simulink model "TestMassAccelerometer_NonlinearModel_LQR_Simulink2017"  (R2018b)
settings: Solver=ode4  StartTime=0.0  StopTime=SIM_TIME  FixedStep=STEP_SIZE  RelTol=1e-3
undefined symbols (not defined in the file): A0, A1, c1, c2, f1, f2, f3, f4, f5, f6, g, Iss, K_lqr_fs, K_lqr_int, m, STEP_TIME, Ts, Vss, x0, x0_int, X_ref, Xss
settings Model: Creator=Roberto  LastModifiedBy=Roberto
settings SFSimCC: SimUseLocalCustomCode=off
settings RTWCC: RTWUseLocalCustomCode=off
settings CodeAppCC: StateflowObjectComments=on

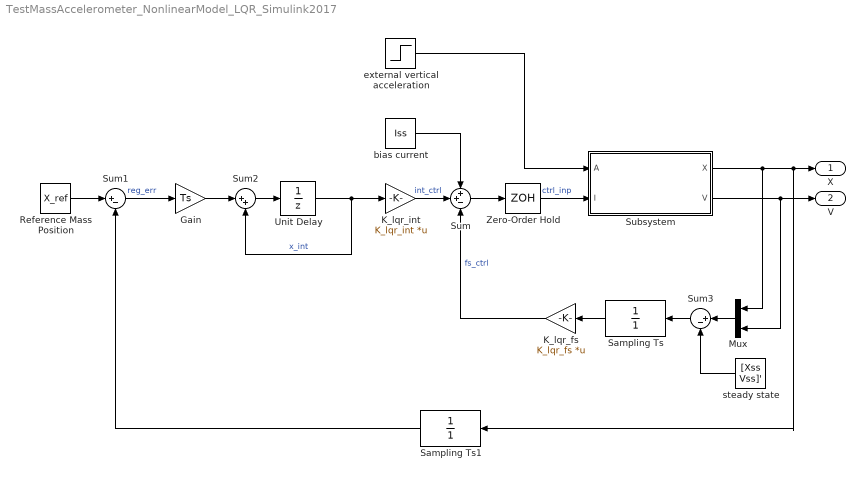
== system TestMassAccelerometer_NonlinearModel_LQR_Simulink2017 ==
  Gain : Gain  Gain=Ts
  K_lqr_fs : Gain  Gain=K_lqr_fs  Multiplication=Matrix(K*u) (u vector)
  K_lqr_int : Gain  Gain=K_lqr_int  Multiplication=Matrix(K*u) (u vector)
  Mux : Mux  Inputs=2
  Reference Mass Position : Constant  Value=X_ref
  Sampling Ts : DiscreteTransferFcn  Denominator=[1]  SampleTime=Ts
  Sampling Ts1 : DiscreteTransferFcn  Denominator=[1]  SampleTime=Ts
  Subsystem : Subsystem
  Sum : Sum  Inputs=++-
  Sum1 : Sum  Inputs=|+-
  Sum2 : Sum  Inputs=|++
  Sum3 : Sum  Inputs=|+-
  Unit Delay : UnitDelay  InitialCondition=x0_int  SampleTime=Ts
  Zero-Order Hold : ZeroOrderHold  SampleTime=Ts
  bias current : Constant  Value=Iss
  external vertical acceleration : Step  Time=STEP_TIME  Before=A0  After=A1  SampleTime=0
  steady state : Constant  Value=[Xss Vss]'
  X : Outport
  V : Outport  Port=2
  wires:
  Zero-Order Hold/1 -> Subsystem/2(I)  "ctrl_inp"
  Subsystem/2(V) -> Mux/2, V/1
  Sampling Ts/1 -> K_lqr_fs/1
  Sum/1 -> Zero-Order Hold/1
  K_lqr_fs/1 -> Sum/3  "fs_ctrl"
  Reference Mass Position/1 -> Sum1/1
  Subsystem/1(X) -> Mux/1, Sampling Ts1/1, X/1
  Sum2/1 -> Unit Delay/1
  Sum1/1 -> Gain/1  "reg_err"
  Unit Delay/1 -> Sum2/2, K_lqr_int/1  "x_int"
  K_lqr_int/1 -> Sum/2  "int_ctrl"
  bias current/1 -> Sum/1
  Sum3/1 -> Sampling Ts/1
  Mux/1 -> Sum3/1
  steady state/1 -> Sum3/2
  external vertical acceleration/1 -> Subsystem/1(A)
  Sampling Ts1/1 -> Sum1/2
  Gain/1 -> Sum2/1

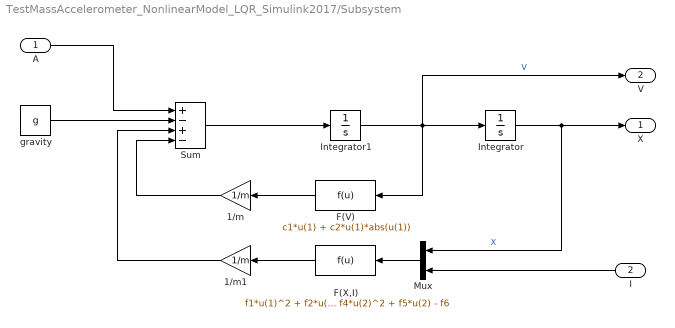
== system TestMassAccelerometer_NonlinearModel_LQR_Simulink2017/Subsystem ==
  A : Inport
  I : Inport  Port=2
  1/m : Gain  Gain=1/m
  1/m1 : Gain  Gain=1/m
  F(V) : Fcn  Expr=c1*u(1) + c2*u(1)*abs(u(1))
  F(X,I) : Fcn  Expr=f1*u(1)^2 + f2*u(1)*u(2) - f3*u(1) + f4*u(2)^2 + f5*u(2) - f6
  Integrator : Integrator  Priority=1  InitialCondition=x0(1)
  Integrator1 : Integrator  Priority=2  InitialCondition=x0(2)
  Mux : Mux  Inputs=2
  Sum : Sum  Inputs=+-+-
  gravity : Constant  Value=g
  X : Outport
  V : Outport  Port=2
  wires:
  I/1 -> Mux/2
  Integrator1/1 -> V/1, Integrator/1, F(V)/1  "V"
  Sum/1 -> Integrator1/1
  gravity/1 -> Sum/2
  A/1 -> Sum/1
  Mux/1 -> F(X,I)/1
  Integrator/1 -> X/1, Mux/1  "X"
  F(X,I)/1 -> 1/m1/1
  F(V)/1 -> 1/m/1
  1/m/1 -> Sum/4
  1/m1/1 -> Sum/3
